simulink model "ADAS_System"  (R2025b)
settings: Solver=VariableStepAuto  StartTime=0.0  StopTime=50  FixedStep=0.1  RelTol=1e-3
undefined symbols (not defined in the file): d_init, fs, v_ego, v_lead
libraries: simulink x3
(part 2 of 2)

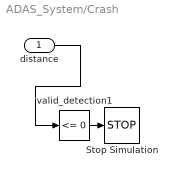
== system ADAS_System/Crash ==
  distance : Inport
  Stop Simulation : Stop
  valid_detection1 : simulink/Logic and Bit Operations/Compare To Constant  relop=<=  const=0  OutDataTypeStr=boolean
  wires:
  valid_detection1/1 -> Stop Simulation/1
  distance/1 -> valid_detection1/1

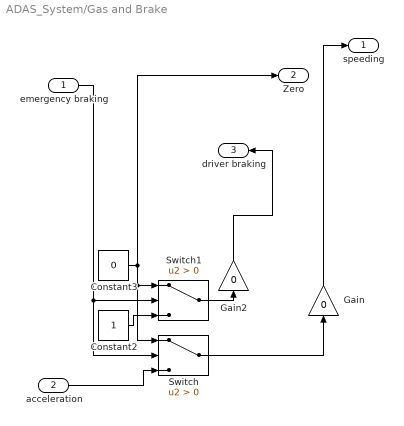
== system ADAS_System/Gas and Brake ==
  emergency braking : Inport
  acceleration : Inport  Port=2
  Constant2 : Constant
  Constant3 : Constant  Value=0
  Gain : Gain  Gain=0
  Gain2 : Gain  Gain=0
  Switch : Switch  Criteria=u2 > Threshold  SaturateOnIntegerOverflow=off  InputSameDT=off
  Switch1 : Switch  Criteria=u2 > Threshold  SaturateOnIntegerOverflow=off  InputSameDT=off
  speeding : Outport
  Zero : Outport  Port=2
  driver braking : Outport  Port=3
  wires:
  Switch1/1 -> Gain2/1
  Constant3/1 -> Zero/1, Switch1/1, Switch/1
  Gain2/1 -> driver braking/1
  Switch/1 -> Gain/1
  emergency braking/1 -> Switch/2, Switch1/2
  acceleration/1 -> Switch/3
  Constant2/1 -> Switch1/3
  Gain/1 -> speeding/1

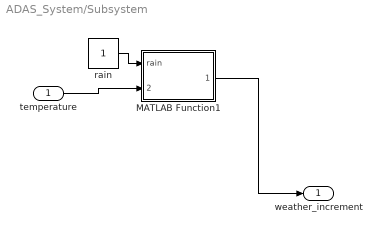
== system ADAS_System/Subsystem ==
  temperature : Inport
  MATLAB Function1 : MATLAB Function  TreatAsAtomicUnit=on
  rain : Constant
  weather_increment : Outport
  wires:
  rain/1 -> MATLAB Function1/1(rain)
  temperature/1 -> MATLAB Function1/2(temperature)
  MATLAB Function1/1(weather_increment) -> weather_increment/1

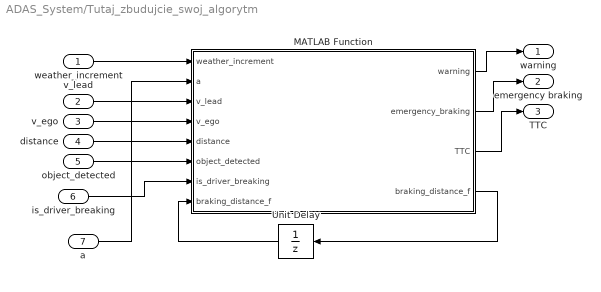
== system ADAS_System/Tutaj_zbudujcie_swoj_algorytm ==
  weather_increment : Inport
  v_lead : Inport  Port=2
  v_ego : Inport  Port=3
  distance : Inport  Port=4
  object_detected : Inport  Port=5
  is_driver_breaking : Inport  Port=6
  a : Inport  Port=7
  MATLAB Function : MATLAB Function  TreatAsAtomicUnit=on
  Unit Delay : UnitDelay  InitialCondition=200  SampleTime=-1  HasFrameUpgradeWarning=on
  warning : Outport
  emergency braking : Outport  Port=2
  "TTC " : Outport  Port=3
  wires:
  MATLAB Function/1(warning) -> warning/1
  MATLAB Function/3(TTC) -> "TTC "/1
  MATLAB Function/2(emergency_braking) -> emergency braking/1
  MATLAB Function/4(braking_distance_f) -> Unit Delay/1
  Unit Delay/1 -> MATLAB Function/8("braking_distance_f ")
  weather_increment/1 -> MATLAB Function/1(weather_increment)
  v_lead/1 -> MATLAB Function/3(v_lead)
  v_ego/1 -> MATLAB Function/4(v_ego)
  distance/1 -> MATLAB Function/5(distance)
  object_detected/1 -> MATLAB Function/6(object_detected)
  is_driver_breaking/1 -> MATLAB Function/7(is_driver_breaking)
  a/1 -> MATLAB Function/2(a)

== matlab function ADAS_System/Tutaj_zbudujcie_swoj_algorytm/MATLAB Function ==
  data: weather_increment input; a input; v_lead input; warning output; v_ego input; distance input; object_detected input; emergency_braking output; TTC output; is_driver_breaking input; braking_distance_f output; braking_distance_f input
function [warning,emergency_braking,TTC,braking_distance_f] = AutonomousEmergencyBraking(weather_increment,a,v_lead,v_ego,distance,object_detected, is_driver_breaking,braking_distance_f)
    if object_detected == false
        warning = 0;
        emergency_braking = 0;
        TTC = 0;
        return
    end

   
    %Zachowanie dystansu w zależności od prędkości i pogody
    %                                  Czas reakcji   Droga hamowania 
    a_max=a + weather_increment;
    preferable_distance_between_cars = v_lead * 0.3 + (v_lead^2)/(2*a_max);
    braking_distance = distance - preferable_distance_between_cars;

    %Filtrowanie szumu z dystansu
    alpha = 0.2;
    braking_distance_f = alpha * braking_distance + (1 - alpha) * braking_distance_f;

    v_rel = v_ego - v_lead;
    %Zabezpieczenie przed ujemną prędkością
    if v_rel <= 0
        TTC = inf;
        TTR = inf;
        TTres = inf;
    else
        TTC = distance / v_rel;
        TTR = braking_distance_f / v_rel;
        %Zmiana czasu na hamowanie w zależności od złej pogody
        
        TTres = v_rel/a_max;
    end

    
    FinTres = TTres + 0.7;
    
    if TTR < FinTres
        warning = 1;
        
        if is_driver_breaking == 0
            emergency_braking = min(1, max(0,(FinTres - TTR) * v_rel) / 10)^2;
        else
            emergency_braking = 0;
        end
    else
        if TTR < (FinTres + 1.0) && TTR >= FinTres
            warning = 1;
            emergency_braking = 0;
        else
            warning = 0;
            emergency_braking = 0;
        end
    end

== matlab function ADAS_System/MATLAB Function ==
  settings: updateMethod=DISCRETE
  data: raw_distance input; clean_distance output; fs input
function clean_distance = radar_filter(raw_distance, fs)
    persistent last_dist;
    
    % Inicjalizacja przy pierwszym kroku symulacji
    if isempty(last_dist)
        last_dist = raw_distance;
    end  
    
    % Obliczenie kroku czasu na podstawie częstotliwości próbkowania
    dt = 1 / fs; 
    
    tau = 0.02; 
    
    % Dynamiczne obliczenie wagi dla nowego pomiaru
    alpha = dt / (tau + dt); 
    
    % Filtracja: waga_nowego * nowy_pomiar + waga_starego * stary_pomiar
    clean_distance = alpha * raw_distance + (1 - alpha) * last_dist;
    
    % Zapisanie obecnej wartości na potrzeby kolejnego kroku
    last_dist = clean_distance;
end

== matlab function ADAS_System/Subsystem/MATLAB Function1 ==
  data: rain input; weather_increment output; temperature input
function weather_increment = fcn(rain, temperature)
    mi_rain=0.4;
    mi_snow=0.2;
    mi_normal=0.7;
    g= 9.81;

    s_breaking_rain=mi_rain*g;
    s_breaking_snow=mi_snow*g;
    s_breaking_normal=mi_normal*g;


    if rain==0
        weather_increment = s_breaking_normal;
    else
        if temperature>0
            weather_increment = s_breaking_rain;
        else
            weather_increment = s_breaking_snow;
        end
    end
